simulink model "prob5"  (R2020b)
settings: Solver=VariableStepAuto  StartTime=0.0  StopTime=10.0  RelTol=1e-3
settings Model: OrderedModelArguments=off  Creator=AVM  LastModifiedBy=AVM

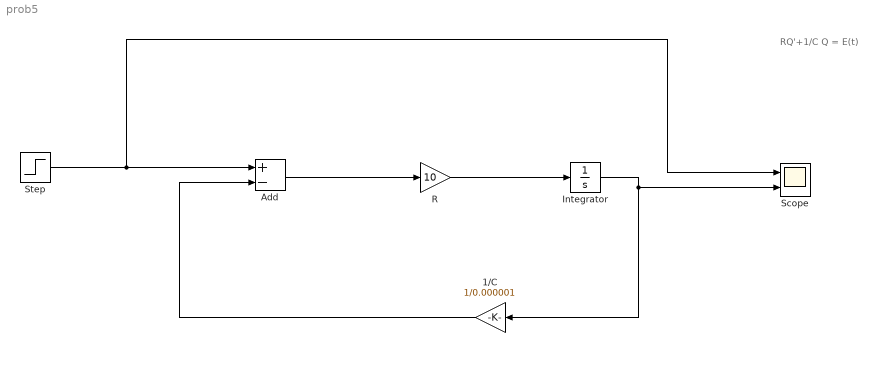
== system prob5 ==
  note: RQ'+1/C Q = E(t)
  1/C : Gain  Gain=1/0.000001
  Add : Sum  Inputs=+-
  Integrator : Integrator
  R : Gain  Gain=10
  Scope : Scope  NumInputPorts=2
  Step : Step  Before=1  After=0  SampleTime=0
  wires:
  Step/1 -> Scope/1, Add/1
  Add/1 -> R/1
  R/1 -> Integrator/1
  Integrator/1 -> 1/C/1, Scope/2
  1/C/1 -> Add/2
